simulink model "Contactor_Control_Standalone"  (R2023b)
settings: Solver=VariableStepAuto  StartTime=0.0  StopTime=10.0  FixedStep=0.001  RelTol=1e-3
settings Model: Creator=mcmas  LastModifiedBy=mcmas

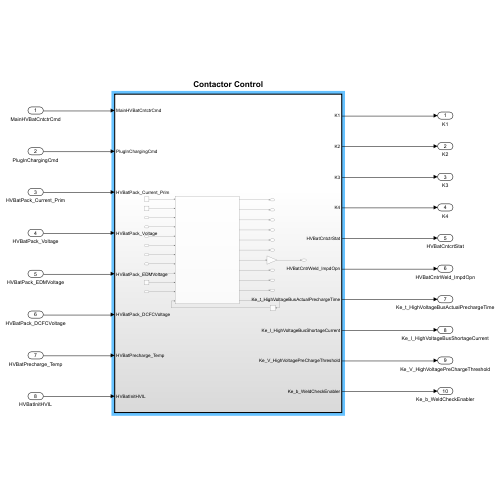
[thumbnail: Simulink's stored preview of the top-level diagram]
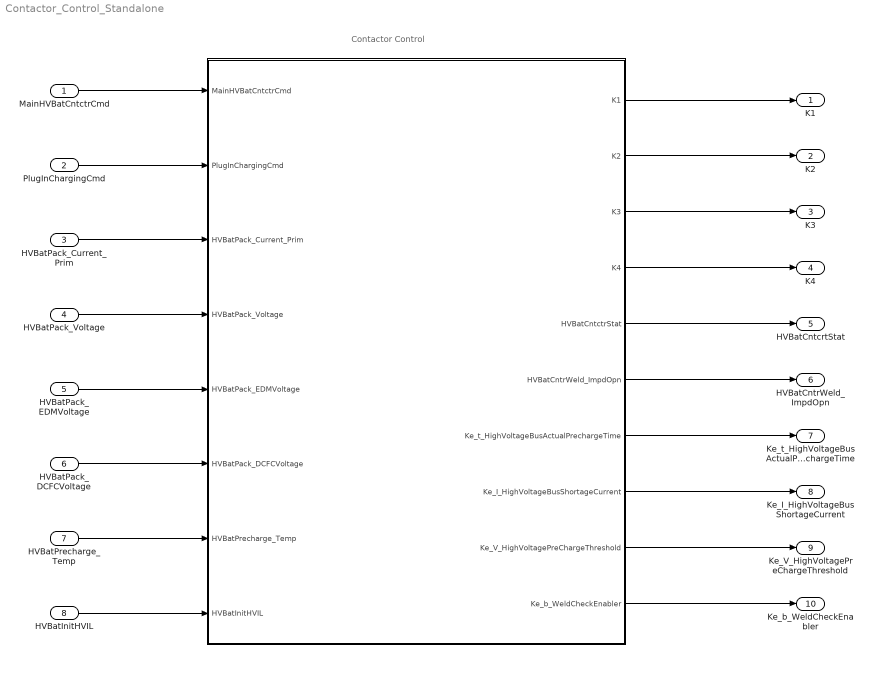
== system Contactor_Control_Standalone ==
  note: Contactor Control
  MainHVBatCntctrCmd : Inport
  PlugInChargingCmd : Inport  Port=2
  HVBatPack_Current_Prim : Inport  Port=3
  HVBatPack_Voltage : Inport  Port=4
  HVBatPack_EDMVoltage : Inport  Port=5
  HVBatPack_DCFCVoltage : Inport  Port=6
  HVBatPrecharge_Temp : Inport  Port=7
  HVBatInitHVIL : Inport  Port=8
  "  " : Subsystem  TreatAsAtomicUnit=on  SystemSampleTime=0.001
  K1 : Outport
  K2 : Outport  Port=2
  K3 : Outport  Port=3
  K4 : Outport  Port=4
  HVBatCntcrtStat : Outport  Port=5
  HVBatCntrWeld_ImpdOpn : Outport  Port=6
  Ke_t_HighVoltageBusActualPrechargeTime : Outport  Port=7
  Ke_I_HighVoltageBusShortageCurrent : Outport  Port=8
  Ke_V_HighVoltagePreChargeThreshold : Outport  Port=9
  Ke_b_WeldCheckEnabler : Outport  Port=10
  wires:
  HVBatPack_DCFCVoltage/1 -> "  "/6(HVBatPack_DCFCVoltage)
  MainHVBatCntctrCmd/1 -> "  "/1(MainHVBatCntctrCmd)
  "  "/5(HVBatCntctrStat) -> HVBatCntcrtStat/1
  HVBatInitHVIL/1 -> "  "/8(HVBatInitHVIL)
  PlugInChargingCmd/1 -> "  "/2(PlugInChargingCmd)
  HVBatPack_Current_Prim/1 -> "  "/3(HVBatPack_Current_Prim)
  HVBatPack_Voltage/1 -> "  "/4(HVBatPack_Voltage)
  "  "/1(K1) -> K1/1
  HVBatPack_EDMVoltage/1 -> "  "/5(HVBatPack_EDMVoltage)
  HVBatPrecharge_Temp/1 -> "  "/7(HVBatPrecharge_Temp)
  "  "/2(K2) -> K2/1
  "  "/3(K3) -> K3/1
  "  "/4(K4) -> K4/1
  "  "/6(HVBatCntrWeld_ImpdOpn) -> HVBatCntrWeld_ImpdOpn/1
  "  "/7(Ke_t_HighVoltageBusActualPrechargeTime) -> Ke_t_HighVoltageBusActualPrechargeTime/1
  "  "/8(Ke_I_HighVoltageBusShortageCurrent) -> Ke_I_HighVoltageBusShortageCurrent/1
  "  "/9(Ke_V_HighVoltagePreChargeThreshold) -> Ke_V_HighVoltagePreChargeThreshold/1
  "  "/10(Ke_b_WeldCheckEnabler) -> Ke_b_WeldCheckEnabler/1

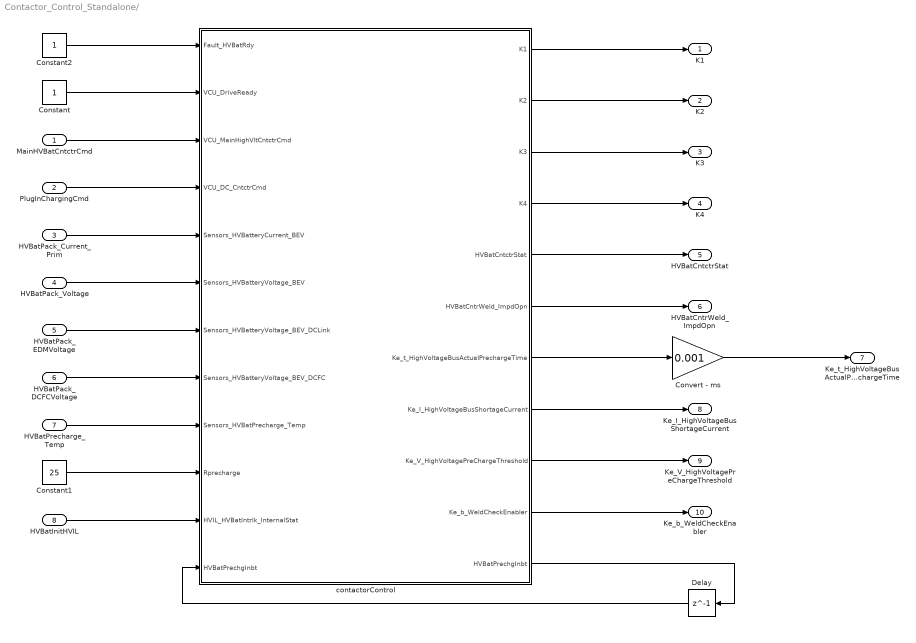
== system Contactor_Control_Standalone/   ==
  MainHVBatCntctrCmd : Inport  SampleTime=0.001
  PlugInChargingCmd : Inport  Port=2  SampleTime=0.001
  HVBatPack_Current_Prim : Inport  Port=3  SampleTime=0.001
  HVBatPack_Voltage : Inport  Port=4  SampleTime=0.001
  HVBatPack_EDMVoltage : Inport  Port=5  SampleTime=0.001
  HVBatPack_DCFCVoltage : Inport  Port=6  SampleTime=0.001
  HVBatPrecharge_Temp : Inport  Port=7
  HVBatInitHVIL : Inport  Port=8
  Constant : Constant
  Constant1 : Constant  Value=25
  Constant2 : Constant
  Convert - ms : Gain  Gain=0.001
  Delay : Delay  DelayLength=1
  contactorControl : MATLAB Function  TreatAsAtomicUnit=on  SystemSampleTime=0.001
  K1 : Outport
  K2 : Outport  Port=2
  K3 : Outport  Port=3
  K4 : Outport  Port=4
  HVBatCntctrStat : Outport  Port=5
  HVBatCntrWeld_ImpdOpn : Outport  Port=6
  Ke_t_HighVoltageBusActualPrechargeTime : Outport  Port=7
  Ke_I_HighVoltageBusShortageCurrent : Outport  Port=8
  Ke_V_HighVoltagePreChargeThreshold : Outport  Port=9
  Ke_b_WeldCheckEnabler : Outport  Port=10
  wires:
  HVBatPack_Current_Prim/1 -> contactorControl/5(Sensors_HVBatteryCurrent_BEV)
  Constant2/1 -> contactorControl/1(Fault_HVBatRdy)
  Constant/1 -> contactorControl/2(VCU_DriveReady)
  MainHVBatCntctrCmd/1 -> contactorControl/3(VCU_MainHighVltCntctrCmd)
  PlugInChargingCmd/1 -> contactorControl/4(VCU_DC_CntctrCmd)
  HVBatPack_Voltage/1 -> contactorControl/6(Sensors_HVBatteryVoltage_BEV)
  HVBatPack_DCFCVoltage/1 -> contactorControl/8(Sensors_HVBatteryVoltage_BEV_DCFC)
  contactorControl/5(HVBatCntctrStat) -> HVBatCntctrStat/1
  HVBatPack_EDMVoltage/1 -> contactorControl/7(Sensors_HVBatteryVoltage_BEV_DCLink)
  HVBatPrecharge_Temp/1 -> contactorControl/9(Sensors_HVBatPrecharge_Temp)
  Constant1/1 -> contactorControl/10(Rprecharge)
  HVBatInitHVIL/1 -> contactorControl/11(HVIL_HVBatIntrlk_InternalStat)
  contactorControl/1(K1) -> K1/1
  contactorControl/2(K2) -> K2/1
  contactorControl/3(K3) -> K3/1
  contactorControl/4(K4) -> K4/1
  contactorControl/6(HVBatCntrWeld_ImpdOpn) -> HVBatCntrWeld_ImpdOpn/1
  contactorControl/7(Ke_t_HighVoltageBusActualPrechargeTime) -> Convert - ms/1
  contactorControl/8(Ke_I_HighVoltageBusShortageCurrent) -> Ke_I_HighVoltageBusShortageCurrent/1
  contactorControl/9(Ke_V_HighVoltagePreChargeThreshold) -> Ke_V_HighVoltagePreChargeThreshold/1
  contactorControl/10(Ke_b_WeldCheckEnabler) -> Ke_b_WeldCheckEnabler/1
  contactorControl/11(HVBatPrechgInbt) -> Delay/1
  Delay/1 -> contactorControl/12("HVBatPrechgInbt ")
  Convert - ms/1 -> Ke_t_HighVoltageBusActualPrechargeTime/1

== matlab function Contactor_Control_Standalone/  /contactorControl ==
  settings: updateMethod=DISCRETE
  data: Fault_HVBatRdy input; VCU_DriveReady input; VCU_MainHighVltCntctrCmd input; VCU_DC_CntctrCmd input; Sensors_HVBatteryCurrent_BEV input; Sensors_HVBatteryVoltage_BEV input; Sensors_HVBatteryVoltage_BEV_DCLink input; Sensors_HVBatteryVoltage_BEV_DCFC input; Sensors_HVBatPrecharge_Temp input; Rprecharge input; HVIL_HVBatIntrlk_InternalStat input; K1 output; HVBatPrechgInbt input; K2 output; K3 output; K4 output; HVBatCntctrStat output; HVBatCntrWeld_ImpdOpn output; Ke_t_HighVoltageBusActualPrechargeTime output; Ke_I_HighVoltageBusShortageCurrent output; Ke_V_HighVoltagePreChargeThreshold output; Ke_b_WeldCheckEnabler output; HVBatPrechgInbt output
function [K1, K2, K3, K4, HVBatCntctrStat, HVBatCntrWeld_ImpdOpn, Ke_t_HighVoltageBusActualPrechargeTime, Ke_I_HighVoltageBusShortageCurrent, Ke_V_HighVoltagePreChargeThreshold, Ke_b_WeldCheckEnabler, HVBatPrechgInbt] = fcn(Fault_HVBatRdy, VCU_DriveReady, VCU_MainHighVltCntctrCmd, VCU_DC_CntctrCmd, Sensors_HVBatteryCurrent_BEV, Sensors_HVBatteryVoltage_BEV, Sensors_HVBatteryVoltage_BEV_DCLink, Sensors_HVBatteryVoltage_BEV_DCFC, Sensors_HVBatPrecharge_Temp, Rprecharge, HVIL_HVBatIntrlk_InternalStat, HVBatPrechgInbt)
%-----------------------------------------------------------
% McMaster Automotive Resource Centre (MARC)
% Electrical Engineer: Romulo Vieira, M.Sc and MBA - PhD Candidate
%-----------------------------------------------------------
% Purpose: Manage precharge relay and contactor sequence with retry + inhibit logic
%-----------------------------------------------------------
% HVBatCntctrStat Mapping:
% 0 – Idle/Waiting
% 1 – Precharge Active
% 2 – Precharge Complete (Main contactors closed)
% 3 – Precharge Failed (necessary cooldown after unique failures of voltage and current)
% 4 – Inhibit State (necessary cooldown after multiple failures)
% 5 - DCFC Charging
% 6 – Contactor Control Shorted High
% 7 - Contactor Control Shorted Low
% VCU_MainHighVltCntctrCmd mapping:
% 0 - open
% 1 - closed
% 2 - impact_open
% 3 - fast_open
% 7 - invalid
% HVBatCntrWeld_ImpdOpn (Contactor welded and has impeded opening when commanded by BPCM) Mapping:
% 0: Normal
% 1: Stuck_Open
% 2: Stuck_Closed
% 3: SNA
% --- Constants ---
Unset_VbusTargetHitIdx             = -1;   % Flag indicating Vbus threshold not yet hit
Min_Samples                        = 0;    % Minimum number of samples where relays and contactor are both active
% Internal Configuration Parameters
Ke_t_PrechargeFailCoolTime             = 1000;   % Cooldown time after one single failed attempt [ms]
Ke_t_ExtraPrechargeFailCoolPenaltyTime = 1000;   % Additional cooldown after two multiple failures [ms]
Ke_t_PrechargeFailMaxPenalty           = 10000;  % Maximum time threshold before enabling precharge inhibit state
Ke_t_BPCM_Precharge_Fail_Penalty_Time  = 15000;  % Hard inhibit time if failures persist [ms]
Ke_I_HighVoltageBusShortageCurrentMin  = 10.8;   % Minimum expected precharge current [A] (Pack current ≥ 0.6 * (pack voltage / Precharge resistance))
                                                 % // max pack voltage = 450 V, Precharge resistance = 25 ohm
Ke_V_HighVoltagePreChargeThreshold     = 0.98 * Sensors_HVBatteryVoltage_BEV;  % Target voltage threshold
Ke_t_HighVoltageBusPrechargeTime       = 100;    % Maximum allowable time for precharging [ms]
Ke_b_WeldCheckEnabler                  = 1;      % Check if weld check diagnostic is enabled (0 - disabled, 1 - enabled)
% --- Persistent Variables ---
persistent I_buffer idx HVBatCntctrStat_Aux VbusTargetHitIdx ...
    t_counter last_PrechargeAllw Prchrgpnltytimer PrechargeFailCount last_HVBatCntctrStat_Aux HVBatCntrWeld_ImpdOpn_Aux Ke_b_WeldCheckEnabler_Aux
if isempty(I_buffer)
    I_buffer               = zeros(Ke_t_HighVoltageBusPrechargeTime,1);
    idx                    = 1;
    HVBatCntctrStat_Aux    = 0;
    VbusTargetHitIdx       = Unset_VbusTargetHitIdx;
    t_counter              = 0;
    last_PrechargeAllw     = 0;
    Prchrgpnltytimer       = 0;
    PrechargeFailCount     = 0; % Represented by k_fail in the flowchart
    last_HVBatCntctrStat_Aux = 0;
    HVBatCntrWeld_ImpdOpn_Aux = 0;
    Ke_b_WeldCheckEnabler_Aux = 1;
end
% --- Default Outputs ---
K1 = 0; K2 = 0; K3 = 0; K4 = 0;
HVBatCntctrStat = HVBatCntctrStat_Aux;
Ke_t_HighVoltageBusActualPrechargeTime = 0;
Ke_I_HighVoltageBusShortageCurrent = 0;
if VCU_MainHighVltCntctrCmd == 3 % VCU_MainHighVltCntctrCmd = 3 means FAST_OPEN
    HVBatCntctrStat_Aux = 0;
end

if VCU_MainHighVltCntctrCmd == 2 % VCU_MainHighVltCntctrCmd = 2 means IMPACT_OPEN
    HVBatCntctrStat_Aux = 0;
    Ke_b_WeldCheckEnabler_Aux = 0;
end

% --- State Machine ---
switch HVBatCntctrStat_Aux
    case 0 % OPEN STATE
        % Set the Battery Contactor States
        K1 = 0; K2 = 0; K3 = 0; K4 = 0;
        % Check Initial conditions
        % HVIL_HVBatIntrlk_InternalStat = 1 (pass),
        % HVIL_HVBatIntrlk_InternalStat = 2 (fail)
        % For precharge initiation HVIL_HVBatIntrlk_InternalStat must pass.
        if VCU_MainHighVltCntctrCmd == 1 && HVBatPrechgInbt == 0 && HVIL_HVBatIntrlk_InternalStat == 1 && Fault_HVBatRdy == 1 && VCU_DriveReady == 1 && Sensors_HVBatPrecharge_Temp < 60
            I_buffer(:) = 0;
            idx = 1;
            VbusTargetHitIdx = Unset_VbusTargetHitIdx;
            t_counter = 0;
            HVBatCntctrStat_Aux = 1;
        end

        %% Shorted High
        
        if VCU_MainHighVltCntctrCmd == 0 && Sensors_HVBatteryVoltage_BEV_DCLink > 270 && Ke_b_WeldCheckEnabler_Aux == 1 
            HVBatCntctrStat_Aux = 6;
            HVBatCntrWeld_ImpdOpn_Aux = 2; 
        end

    case 1  % PRECHARGING STATE
        % Abort if initial conditions are no longer valid
        if VCU_MainHighVltCntctrCmd == 0 || HVBatPrechgInbt == 1 || HVIL_HVBatIntrlk_InternalStat == 2 || Fault_HVBatRdy == 0 || VCU_DriveReady == 0 || Sensors_HVBatPrecharge_Temp >= 60
            HVBatCntctrStat_Aux = 0;
        end
        % Set precharge relays ON
        K1 = 0; K2 = 1; K3 = 1; K4 = 0;
        %
        % if Fault_K1_Shorted_Low_Condition == 1
        %     HVBatCntctrStat_Aux = 7; % K1 Shorted Low
        % end
        % if Fault_K4_Shorted_Low_Condition == 1
        %     HVBatCntctrStat_Aux = 7; % K4 Shorted Low
        % end
        % Record current
        if t_counter == 0
            I_buffer(idx) = Sensors_HVBatteryVoltage_BEV / Rprecharge;
        else
            I_buffer(idx) = Sensors_HVBatteryCurrent_BEV;
        end
        Ke_I_HighVoltageBusShortageCurrent = max(I_buffer);
        % Voltage target check
        if VbusTargetHitIdx == Unset_VbusTargetHitIdx && Sensors_HVBatteryVoltage_BEV_DCLink >= Ke_V_HighVoltagePreChargeThreshold
            VbusTargetHitIdx = t_counter + 1;
        end
        % Time since start or since target hit
        if VbusTargetHitIdx ~= Unset_VbusTargetHitIdx
            delta_samples = VbusTargetHitIdx;
        else
            delta_samples = t_counter;
        end
        % SUCCESS - PRECHARGE CONDITIONS ARE MET
        if t_counter < Ke_t_HighVoltageBusPrechargeTime && ...
                VbusTargetHitIdx ~= Unset_VbusTargetHitIdx && delta_samples < Ke_t_HighVoltageBusPrechargeTime && Ke_I_HighVoltageBusShortageCurrent >= Ke_I_HighVoltageBusShortageCurrentMin
            
            % Set the next Battery Contactor Status
            HVBatCntctrStat_Aux = 2;
            % Set the Battery Contactor States
            K1 = 1; K2 = 0; K3 = 0; K4 = 0;
            PrechargeFailCount = 0;
            Prchrgpnltytimer = 0;
        % FAILURE - PRECHARGE CONDITIONS ARE NOT MET
        elseif t_counter == Ke_t_HighVoltageBusPrechargeTime && ...
               (VbusTargetHitIdx == Unset_VbusTargetHitIdx || delta_samples == Ke_t_HighVoltageBusPrechargeTime || Ke_I_HighVoltageBusShortageCurrent < Ke_I_HighVoltageBusShortageCurrentMin)
            % Set the Battery Contactor States
            K1 = 0; K2 = 0; K3 = 0; K4 = 0;
           % Set the Battery Contactor Status
            HVBatCntctrStat_Aux = 3;
            % Update the total cooling time before re-attempt
            PrechargeFailCount = PrechargeFailCount + 1;
            Prchrgpnltytimer = Prchrgpnltytimer + Ke_t_PrechargeFailCoolTime;
            if PrechargeFailCount >= 2
                Prchrgpnltytimer = Ke_t_ExtraPrechargeFailCoolPenaltyTime;
            end
            if PrechargeFailCount >= 10
                HVBatCntctrStat_Aux = 4;
                HVBatPrechgInbt = 1;
                Prchrgpnltytimer = Ke_t_BPCM_Precharge_Fail_Penalty_Time;
            end
        end
        % Update counters
        t_counter = t_counter + 1;
        idx = idx + 1;
        if idx > Ke_t_HighVoltageBusPrechargeTime, idx = 1; end
    case 2  % PRECHARGE COMPLETE OR CLOSED
        % Set the Battery Contactor States
        K1 = 1; K2 = 0; K3 = 0; K4 = 0;
        % If statement to detect DCFC charging
        if VCU_DC_CntctrCmd == 1
            HVBatCntctrStat_Aux = 5; % DCFC CHARGING
        end
        if VCU_MainHighVltCntctrCmd == 0
            HVBatCntctrStat_Aux = 0;
        end

        if VCU_MainHighVltCntctrCmd == 1 && Sensors_HVBatteryVoltage_BEV_DCLink < 270 && Ke_b_WeldCheckEnabler_Aux == 1
            HVBatCntctrStat_Aux = 7;
            HVBatCntrWeld_ImpdOpn_Aux = 1;
        end

    case 3 % FAULT: PRECHARGE FAILED STATE 4 --> 3
        % Set the Battery Contactor States
        K1 = 0; K2 = 0; K3 = 0; K4 = 0;
        if Prchrgpnltytimer > 0
            Prchrgpnltytimer = Prchrgpnltytimer - 1;
        else
            HVBatCntctrStat_Aux = 0;
        end
    case 4  % FAULT: PRECHARGE INHIBIT STATE - 5 -- > 4
        % Set the Battery Contactor States
        K1 = 0; K2 = 0; K3 = 0; K4 = 0;
        if Prchrgpnltytimer > 0
            Prchrgpnltytimer = Prchrgpnltytimer - 1;
        else
            Prchrgpnltytimer = 0;
            HVBatPrechgInbt = 0;
            HVBatCntctrStat_Aux = 0;
            PrechargeFailCount = 0;
        end
    case 5 % DCFC CHARGING
        % Set the Battery Contactor States
        K1 = 1; K2 = 0; K3 = 0; K4 = 1;
        if VCU_DC_CntctrCmd == 0
            if VCU_MainHighVltCntctrCmd == 0
                HVBatCntctrStat_Aux = 0; % switch to OPEN
            else
                HVBatCntctrStat_Aux = 2; % switch to CLOSED
            end
        end
    
    case 6 % FAULT: Shorted High
       
        if VCU_MainHighVltCntctrCmd == 0 && Sensors_HVBatteryVoltage_BEV_DCLink < 270
            HVBatCntctrStat_Aux = 0;
            HVBatCntrWeld_ImpdOpn_Aux = 0;
        end

    case 7 % FAULT: Shorted Low

        if VCU_DC_CntctrCmd == 0 && Sensors_HVBatteryVoltage_BEV_DCFC < 270 && VCU_MainHighVltCntctrCmd == 1 && Sensors_HVBatteryVoltage_BEV_DCLink > 270
            HVBatCntctrStat_Aux = 2;
            HVBatCntrWeld_ImpdOpn_Aux = 0;
        end
    otherwise
        K1 = 0; K2 = 0; K3 = 0; K4 = 0;
        HVBatCntctrStat_Aux = 0;
end
% --- Final Outputs ---
HVBatCntctrStat = HVBatCntctrStat_Aux;
HVBatCntrWeld_ImpdOpn = HVBatCntrWeld_ImpdOpn_Aux;
Ke_b_WeldCheckEnabler = Ke_b_WeldCheckEnabler_Aux;
Ke_t_HighVoltageBusActualPrechargeTime = max(0, VbusTargetHitIdx + ...
    Min_Samples * (VbusTargetHitIdx ~= Unset_VbusTargetHitIdx));
last_PrechargeAllw = double(Fault_HVBatRdy);
last_HVBatCntctrStat_Aux = HVBatCntctrStat_Aux;
end
